simulink model "T2_unstable_gain_me23b201"  (R2025a)
settings: Solver=VariableStepAuto  StartTime=0.0  StopTime=10.0  RelTol=1e-3
undefined symbols (not defined in the file or in its folder): Gm
settings Model: Creator=abhi  LastModifiedBy=abhi

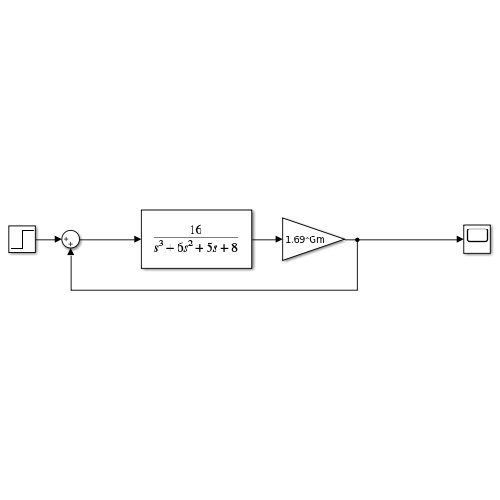
[thumbnail: Simulink's stored preview of the top-level diagram]
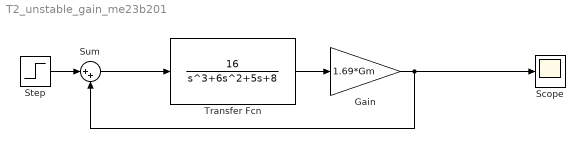
== system T2_unstable_gain_me23b201 ==
  Gain : Gain  Gain=1.69*Gm
  Scope : Scope
      settings: ActiveDisplayYMinimum=-1.4199272179774896E+6  ActiveDisplayYMaximum=2.6945448438542583E+6
  Step : Step  SampleTime=0
  Sum : Sum  Inputs=|++
  Transfer Fcn : TransferFcn  Numerator=[16]  Denominator=[1 6 5 8]
  wires:
  Transfer Fcn/1 -> Gain/1
  Gain/1 -> Sum/2, Scope/1
  Step/1 -> Sum/1
  Sum/1 -> Transfer Fcn/1
